simulink model "main"  (R2022a)
settings: Solver=FixedStepDiscrete  StartTime=0.0  StopTime=Inf  FixedStep=(50e-6)-(sim_en*4.995e-5)  RelTol=1e-3  EnableMultiTasking=on
model workspace (MAT data in the model file):
  Param : Simulink.Parameter (value not decoded)
  ac_ok : Simulink.Signal (value not decoded)
  ac_ok_120 : Simulink.Signal (value not decoded)
  bulk_voltage : Simulink.Signal (value not decoded)
  burstduty_integ_max : Simulink.Signal (value not decoded)
  burstduty_integ_min : Simulink.Signal (value not decoded)
  burstduty_ki : Simulink.Signal (value not decoded)
  burstduty_kp : Simulink.Signal (value not decoded)
  calib_ok : Simulink.Signal (value not decoded)
  can_addr1 : Simulink.Signal (value not decoded)
  can_addr2 : Simulink.Signal (value not decoded)
  can_addr3 : Simulink.Signal (value not decoded)
  can_addr4 : Simulink.Signal (value not decoded)
  can_data_rx : Simulink.Signal (value not decoded)
  can_data_tx : Simulink.Signal (value not decoded)
  can_timeout_120 : Simulink.Signal (value not decoded)
  chksum_scircv : Simulink.Signal (value not decoded)
  clllc_en_120 : Simulink.Signal (value not decoded)
  clllc_fault_120 : Simulink.Signal (value not decoded)
  clllc_ok_120 : Simulink.Signal (value not decoded)
  cmpss1h : Simulink.Signal (value not decoded)
  cmpss1l : Simulink.Signal (value not decoded)
  cmpss2h : Simulink.Signal (value not decoded)
  cmpss2l : Simulink.Signal (value not decoded)
  cmpss3h : Simulink.Signal (value not decoded)
  cmpss3l : Simulink.Signal (value not decoded)
  cmpss4h : Simulink.Signal (value not decoded)
  cmpss4l : Simulink.Signal (value not decoded)
  cmpss5h : Simulink.Signal (value not decoded)
  cmpss5l : Simulink.Signal (value not decoded)
  cmpss6h : Simulink.Signal (value not decoded)
  cmpss6l : Simulink.Signal (value not decoded)
  cmpss7h : Simulink.Signal (value not decoded)
  cmpss7l : Simulink.Signal (value not decoded)
  cmpss8h : Simulink.Signal (value not decoded)
  cmpss8l : Simulink.Signal (value not decoded)
  cnt_idle : Simulink.Signal (value not decoded)
  cnt_orps : Simulink.Signal (value not decoded)
  cnt_scircv : Simulink.Signal (value not decoded)
  cnt_scixmt : Simulink.Signal (value not decoded)
  cnt_scixmt_func : Simulink.Signal (value not decoded)
  cnt_temp_mux : Simulink.Signal (value not decoded)
  cnt_vdroop : Simulink.Signal (value not decoded)
  config_ok : Simulink.Signal (value not decoded)
  control_en : Simulink.Signal (value not decoded)
  cp_ready_120 : Simulink.Signal (value not decoded)
  d2d_en : Simulink.Signal (value not decoded)
  dchg_off : Simulink.Signal (value not decoded)
  debug_dacb : Simulink.Signal (value not decoded)
  debug_dacc : Simulink.Signal (value not decoded)
  debug_msg1 : Simulink.Signal (value not decoded)
  debug_msg2 : Simulink.Signal (value not decoded)
  debug_msg3 : Simulink.Signal (value not decoded)
  debug_msg4 : Simulink.Signal (value not decoded)
  debug_msg5 : Simulink.Signal (value not decoded)
  debug_msg6 : Simulink.Signal (value not decoded)
  dir_v2g : Simulink.Signal (value not decoded)
  eoss_llc1 : Simulink.Signal (value not decoded)
  eoss_llc2 : Simulink.Signal (value not decoded)
  eoss_orps : Simulink.Signal (value not decoded)
  fault_ocp : Simulink.Signal (value not decoded)
  fault_otp : Simulink.Signal (value not decoded)
  fault_ovp : Simulink.Signal (value not decoded)
  fut_en : Simulink.Signal (value not decoded)
  fwd_en_120 : Simulink.Signal (value not decoded)
  gain_llc1_sec_idc : Simulink.Signal (value not decoded)
  gain_llc1_temp_sr : Simulink.Signal (value not decoded)
  gain_llc2_sec_idc : Simulink.Signal (value not decoded)
  gain_vbat : Simulink.Signal (value not decoded)
  gain_vbulk : Simulink.Signal (value not decoded)
  gain_vout : Simulink.Signal (value not decoded)
  input_current_phasea : Simulink.Signal (value not decoded)
  input_current_phaseb : Simulink.Signal (value not decoded)
  input_current_phasec : Simulink.Signal (value not decoded)
  input_freq : Simulink.Signal (value not decoded)
  input_power : Simulink.Signal (value not decoded)
  input_voltage_phasea : Simulink.Signal (value not decoded)
  input_voltage_phaseb : Simulink.Signal (value not decoded)
  input_voltage_phasec : Simulink.Signal (value not decoded)
  ishare_arbiter : Simulink.Signal (value not decoded)
  ishare_thresh : Simulink.Signal (value not decoded)
  led_g : Simulink.Signal (value not decoded)
  led_r : Simulink.Signal (value not decoded)
  led_y : Simulink.Signal (value not decoded)
  llc1_burst_integ : Simulink.Signal (value not decoded)
  llc1_burstduty_buffer : Simulink.Signal (value not decoded)
  llc1_pfm_error : Simulink.Signal (value not decoded)
  llc1_pfm_integ : Simulink.Signal (value not decoded)
  llc1_pfm_prop : Simulink.Signal (value not decoded)
  llc1_pri_idc : Simulink.Signal (value not decoded)
  llc1_ps_buffer : Simulink.Signal (value not decoded)
  llc1_pspwm_error : Simulink.Signal (value not decoded)
  llc1_pspwm_integ : Simulink.Signal (value not decoded)
  llc1_pspwm_prop : Simulink.Signal (value not decoded)
  llc1_sec_idc : Simulink.Signal (value not decoded)
  llc1_temp_sr : Simulink.Signal (value not decoded)
  llc1_ts_tbctr_buffer : Simulink.Signal (value not decoded)
  llc2_burst_integ : Simulink.Signal (value not decoded)
  llc2_burstduty_buffer : Simulink.Signal (value not decoded)
  llc2_en : Simulink.Signal (value not decoded)
  llc2_en_buffer : Simulink.Signal (value not decoded)
  llc2_pfm_error : Simulink.Signal (value not decoded)
  llc2_pfm_integ : Simulink.Signal (value not decoded)
  llc2_pfm_prop : Simulink.Signal (value not decoded)
  llc2_pri_idc : Simulink.Signal (value not decoded)
  llc2_ps_buffer : Simulink.Signal (value not decoded)
  llc2_pspwm_error : Simulink.Signal (value not decoded)
  llc2_pspwm_integ : Simulink.Signal (value not decoded)
  llc2_pspwm_prop : Simulink.Signal (value not decoded)
  llc2_sec_idc : Simulink.Signal (value not decoded)
  llc2_temp_sr : Simulink.Signal (value not decoded)
  llc2_ts_tbctr_buffer : Simulink.Signal (value not decoded)
  loop_adcint : Simulink.Signal (value not decoded)
  loop_control : Simulink.Signal (value not decoded)
  loop_idle : Simulink.Signal (value not decoded)
  mid_bulk_voltage : Simulink.Signal (value not decoded)
  mode_120 : Simulink.Signal (value not decoded)
  mode_cc_cv : Simulink.Signal (value not decoded)
  myParam : mpt.Parameter (value not decoded)
  obc_ok_120 : Simulink.Signal (value not decoded)
  offset_llc1_sec_idc : Simulink.Signal (value not decoded)
  offset_llc1_temp_sr : Simulink.Signal (value not decoded)
  offset_llc2_sec_idc : Simulink.Signal (value not decoded)
  offset_vbat : Simulink.Signal (value not decoded)
  offset_vbulk : Simulink.Signal (value not decoded)
  offset_vout : Simulink.Signal (value not decoded)
  openloop_en : Simulink.Signal (value not decoded)
  openloop_fault_en : Simulink.Signal (value not decoded)
  ot_fault_120 : Simulink.Signal (value not decoded)
  pfc_en : Simulink.Signal (value not decoded)
  pfc_en_120 : Simulink.Signal (value not decoded)
  pfc_fw_revision : Simulink.Signal (value not decoded)
  pfc_fw_revision_bootloader : Simulink.Signal (value not decoded)
  pfc_fw_revision_debug : Simulink.Signal (value not decoded)
  pfc_ok : Simulink.Signal (value not decoded)
  pfc_ok_120 : Simulink.Signal (value not decoded)
  pfm_a0 : Simulink.Signal (value not decoded)
  pfm_a1 : Simulink.Signal (value not decoded)
  pfm_integ_max : Simulink.Signal (value not decoded)
  pfm_integ_min : Simulink.Signal (value not decoded)
  pfm_ki : Simulink.Signal (value not decoded)
  pfm_kp : Simulink.Signal (value not decoded)
  pri_fut_en : Simulink.Signal (value not decoded)
  pri_fut_en_buffer : Simulink.Signal (value not decoded)
  pri_halfbridge_en : Simulink.Signal (value not decoded)
  pri_halfbridge_en_buffer : Simulink.Signal (value not decoded)
  pspwm_integ_max : Simulink.Signal (value not decoded)
  pspwm_integ_min : Simulink.Signal (value not decoded)
  pspwm_ki : Simulink.Signal (value not decoded)
  pspwm_kp : Simulink.Signal (value not decoded)
  ref_idclink_max : Simulink.Signal (value not decoded)
  ref_iout : Simulink.Signal (value not decoded)
  ref_iout_calib : Simulink.Signal (value not decoded)
  ref_iout_llc1 : Simulink.Signal (value not decoded)
  ref_iout_llc1_calib : Simulink.Signal (value not decoded)
  ref_iout_llc2 : Simulink.Signal (value not decoded)
  ref_iout_llc2_calib : Simulink.Signal (value not decoded)
  ref_pout : Simulink.Signal (value not decoded)
  ref_ss_llc1 : Simulink.Signal (value not decoded)
  ref_ss_llc2 : Simulink.Signal (value not decoded)
  ref_ss_orps : Simulink.Signal (value not decoded)
  ref_vbat : Simulink.Signal (value not decoded)
  ref_vbat_calib : Simulink.Signal (value not decoded)
  ref_vbulk : Simulink.Signal (value not decoded)
  ref_vbulk_calib : Simulink.Signal (value not decoded)
  ref_vbulk_llc1_calib : Simulink.Signal (value not decoded)
  ref_vbulk_llc2_calib : Simulink.Signal (value not decoded)
  ref_vout : Simulink.Signal (value not decoded)
  ref_vout_calib : Simulink.Signal (value not decoded)
  relay_en : Simulink.Signal (value not decoded)
  reset_flag : Simulink.Signal (value not decoded)
  rev_en_120 : Simulink.Signal (value not decoded)
  runtime_control : Simulink.Signal (value not decoded)
  runtime_idle : Simulink.Signal (value not decoded)
  scircv_buffer : Simulink.Signal (value not decoded)
  scircv_buffer_tmp : Simulink.Signal (value not decoded)
  scircv_buffer_tmp_idx0 : Simulink.Signal (value not decoded)
  scircv_chksum : Simulink.Signal (value not decoded)
  scircv_chksum_ok : Simulink.Signal (value not decoded)
  scircv_parse_ok : Simulink.Signal (value not decoded)
  scixmt_buffer : Simulink.Signal (value not decoded)
  scixmt_chksum : Simulink.Signal (value not decoded)
  scixmt_func : Simulink.Signal (value not decoded)
  scixmt_word0_lsb : Simulink.Signal (value not decoded)
  scixmt_word0_msb : Simulink.Signal (value not decoded)
  scixmt_word1_lsb : Simulink.Signal (value not decoded)
  scixmt_word1_msb : Simulink.Signal (value not decoded)
  scixmt_word2_lsb : Simulink.Signal (value not decoded)
  scixmt_word2_msb : Simulink.Signal (value not decoded)
  scixmt_wr : Simulink.Signal (value not decoded)
  ss_step : Simulink.Signal (value not decoded)
  state_calib : Simulink.Signal (value not decoded)
  state_control : Simulink.Signal (value not decoded)
  state_hkeep : Simulink.Signal (value not decoded)
  status_cmpss : Simulink.Signal (value not decoded)
  status_control : Simulink.Signal (value not decoded)
  status_digin : Simulink.Signal (value not decoded)
  status_digout : Simulink.Signal (value not decoded)
  status_fault : Simulink.Signal (value not decoded)
  status_input : Simulink.Signal (value not decoded)
  status_pfc : Simulink.Signal (value not decoded)
  temp_inlet : Simulink.Signal (value not decoded)
  temp_llc1_fet_hs : Simulink.Signal (value not decoded)
  temp_llc2_fet_hs : Simulink.Signal (value not decoded)
  temp_mux : Simulink.Signal (value not decoded)
  temp_mux_s0 : Simulink.Signal (value not decoded)
  temp_mux_s1 : Simulink.Signal (value not decoded)
  temp_mux_s2 : Simulink.Signal (value not decoded)
  temp_outlet : Simulink.Signal (value not decoded)
  temp_pfc_fet_hsa : Simulink.Signal (value not decoded)
  temp_pfc_fet_hsb : Simulink.Signal (value not decoded)
  temp_pfc_fet_hsc : Simulink.Signal (value not decoded)
  temp_pfc_fet_lsa : Simulink.Signal (value not decoded)
  temp_pfc_fet_lsb : Simulink.Signal (value not decoded)
  temp_pfc_fet_lsc : Simulink.Signal (value not decoded)
  test_mode : Simulink.Signal (value not decoded)
  tfcv_cc : Simulink.Signal (value not decoded)
  tfcv_cc_llc2 : Simulink.Signal (value not decoded)
  tfcv_cv : Simulink.Signal (value not decoded)
  tfcv_sr_en : Simulink.Signal (value not decoded)
  tfv_assert_llc1_pri_idc : Simulink.Signal (value not decoded)
  tfv_assert_llc1_sec_idc : Simulink.Signal (value not decoded)
  tfv_assert_llc1_temp_sr : Simulink.Signal (value not decoded)
  tfv_assert_llc2_pri_idc : Simulink.Signal (value not decoded)
  tfv_assert_llc2_sec_idc : Simulink.Signal (value not decoded)
  tfv_assert_llc2_temp_sr : Simulink.Signal (value not decoded)
  tfv_assert_temp_outlet : Simulink.Signal (value not decoded)
  tfv_assert_vaux_uv : Simulink.Signal (value not decoded)
  tfv_assert_vbat : Simulink.Signal (value not decoded)
  tfv_assert_vbulk : Simulink.Signal (value not decoded)
  tfv_assert_vout : Simulink.Signal (value not decoded)
  tfv_cnt_tz : Simulink.Signal (value not decoded)
  tfv_deassert_llc1_pri_idc : Simulink.Signal (value not decoded)
  tfv_deassert_llc1_sec_idc : Simulink.Signal (value not decoded)
  tfv_deassert_llc1_temp_sr : Simulink.Signal (value not decoded)
  tfv_deassert_llc2_pri_idc : Simulink.Signal (value not decoded)
  tfv_deassert_llc2_sec_idc : Simulink.Signal (value not decoded)
  tfv_deassert_llc2_temp_sr : Simulink.Signal (value not decoded)
  tfv_deassert_temp_outlet : Simulink.Signal (value not decoded)
  tfv_deassert_vaux_uv : Simulink.Signal (value not decoded)
  tfv_deassert_vbat : Simulink.Signal (value not decoded)
  tfv_deassert_vbulk : Simulink.Signal (value not decoded)
  tfv_deassert_vout : Simulink.Signal (value not decoded)
  tfv_llc1_pri_idc : Simulink.Signal (value not decoded)
  tfv_llc1_sec_idc : Simulink.Signal (value not decoded)
  tfv_llc1_temp_sr : Simulink.Signal (value not decoded)
  tfv_llc2_pri_idc : Simulink.Signal (value not decoded)
  tfv_llc2_sec_idc : Simulink.Signal (value not decoded)
  tfv_llc2_temp_sr : Simulink.Signal (value not decoded)
  tfv_temp_outlet : Simulink.Signal (value not decoded)
  tfv_vaux_uv : Simulink.Signal (value not decoded)
  tfv_vbat : Simulink.Signal (value not decoded)
  tfv_vbulk : Simulink.Signal (value not decoded)
  tfv_vout : Simulink.Signal (value not decoded)
  timer_1ms : Simulink.Signal (value not decoded)
  tz : Simulink.Signal (value not decoded)
  valve_en : Simulink.Signal (value not decoded)
  vaux : Simulink.Signal (value not decoded)
  vbat : Simulink.Signal (value not decoded)
  vbulk : Simulink.Signal (value not decoded)
  vout : Simulink.Signal (value not decoded)
undefined symbols (not defined in the file or in its folder): CAN_O_INT, CANA_BASE, Down, GPTRIP1SEL, GPTRIP2SEL, TZ1, TZ2, Up
libraries: hdlsllib x159, simulink x100, c2837xDlib x24, c2807xlib x16, c280xlib x13, c2802xlib x12, canmsglib x8, idelinklib_common x2, c2000lib x1, c281xlib x1
(part 5 of 15)

== system main/Task_Manager/Tmr_1mS/codegen/Task_1mS/GPIO_Handler ==
  function : TriggerPort  TriggerType=function-call  VariantControl=Variant
  Cast{,1..3} (4 alike) : DataTypeConversion  OutDataTypeStr=boolean  SaturateOnIntegerOverflow=off  RndMeth=Floor
  Cast{4..7} (4 alike) : DataTypeConversion  Commented=on  OutDataTypeStr=boolean  SaturateOnIntegerOverflow=off  RndMeth=Floor
  Constant : Constant
  Constant1 : Constant  Commented=on
  Data Store Read1 : DataStoreRead  Commented=on  DataStoreName=pfc_en_120  IndexOptions=Index vector (dialog)  Indices=1  OutputSizes=1
  Data Store Read2 : DataStoreRead  Commented=on  DataStoreName=obc_ok_120  IndexOptions=Index vector (dialog)  Indices=1  OutputSizes=1
  Data Store Read5 : DataStoreRead  Commented=on  DataStoreName=clllc_ok_120  IndexOptions=Index vector (dialog)  Indices=1  OutputSizes=1
  Data Store Write1 : DataStoreWrite  DataStoreName=ac_ok_120  IndexOptions=Index vector (dialog)  Indices=1  OutputSizes=1
  Data Store Write12 : DataStoreWrite  DataStoreName=cp_ready_120  IndexOptions=Index vector (dialog)  Indices=1  OutputSizes=1
  Data Store Write2 : DataStoreWrite  DataStoreName=pfc_ok_120  IndexOptions=Index vector (dialog)  Indices=1  OutputSizes=1
  Data Store Write3 : DataStoreWrite  DataStoreName=clllc_en_120  IndexOptions=Index vector (dialog)  Indices=1  OutputSizes=1
  Digital Input1 : c2837xDlib/Digital Input  Commented=on  GPIO_Number=GPIO56~GPIO63  GPIO_Bit0=off  GPIO_Bit1=off  GPIO_Bit2=off  GPIO_Bit3=off  GPIO_Bit4=on  GPIO_Bit5=off  GPIO_Bit6=off  GPIO_Bit7=off  sampleTime=0.001  dataType=auto  GPIO_Bit0_Qualification=Sync to SYSCLKOUT  GPIO_Bit1_Qualification=Sync to SYSCLKOUT  GPIO_Bit2_Qualification=Sync to SYSCLKOUT  GPIO_Bit3_Qualification=Sync to SYSCLKOUT  GPIO_Bit4_Qualification=Sync to SYSCLKOUT  GPIO_Bit5_Qualification=Sync to SYSCLKOUT  GPIO_Bit6_Qualification=Sync to SYSCLKOUT  GPIO_Bit7_Qualification=Sync to SYSCLKOUT  Qualification_Period=-1
      settings: SourceProductBaseCode=TIC2000
  Digital Input2 : c2837xDlib/Digital Input  Commented=on  GPIO_Number=GPIO56~GPIO63  GPIO_Bit0=off  GPIO_Bit1=off  GPIO_Bit2=off  GPIO_Bit3=on  GPIO_Bit4=off  GPIO_Bit5=off  GPIO_Bit6=off  GPIO_Bit7=off  sampleTime=0.001  dataType=auto  GPIO_Bit0_Qualification=Sync to SYSCLKOUT  GPIO_Bit1_Qualification=Sync to SYSCLKOUT  GPIO_Bit2_Qualification=Sync to SYSCLKOUT  GPIO_Bit3_Qualification=Sync to SYSCLKOUT  GPIO_Bit4_Qualification=Sync to SYSCLKOUT  GPIO_Bit5_Qualification=Sync to SYSCLKOUT  GPIO_Bit6_Qualification=Sync to SYSCLKOUT  GPIO_Bit7_Qualification=Sync to SYSCLKOUT  Qualification_Period=-1
      settings: SourceProductBaseCode=TIC2000
  Digital Input3 : c2837xDlib/Digital Input  Commented=on  GPIO_Number=GPIO56~GPIO63  GPIO_Bit0=off  GPIO_Bit1=on  GPIO_Bit2=off  GPIO_Bit3=off  GPIO_Bit4=off  GPIO_Bit5=off  GPIO_Bit6=off  GPIO_Bit7=off  sampleTime=0.001  dataType=auto  GPIO_Bit0_Qualification=Sync to SYSCLKOUT  GPIO_Bit1_Qualification=Sync to SYSCLKOUT  GPIO_Bit2_Qualification=Sync to SYSCLKOUT  GPIO_Bit3_Qualification=Sync to SYSCLKOUT  GPIO_Bit4_Qualification=Sync to SYSCLKOUT  GPIO_Bit5_Qualification=Sync to SYSCLKOUT  GPIO_Bit6_Qualification=Sync to SYSCLKOUT  GPIO_Bit7_Qualification=Sync to SYSCLKOUT  Qualification_Period=-1
      settings: SourceProductBaseCode=TIC2000
  Digital Input4 : c2837xDlib/Digital Input  Commented=on  GPIO_Number=GPIO56~GPIO63  GPIO_Bit0=off  GPIO_Bit1=off  GPIO_Bit2=on  GPIO_Bit3=off  GPIO_Bit4=off  GPIO_Bit5=off  GPIO_Bit6=off  GPIO_Bit7=off  sampleTime=0.001  dataType=auto  GPIO_Bit0_Qualification=Sync to SYSCLKOUT  GPIO_Bit1_Qualification=Sync to SYSCLKOUT  GPIO_Bit2_Qualification=Sync to SYSCLKOUT  GPIO_Bit3_Qualification=Sync to SYSCLKOUT  GPIO_Bit4_Qualification=Sync to SYSCLKOUT  GPIO_Bit5_Qualification=Sync to SYSCLKOUT  GPIO_Bit6_Qualification=Sync to SYSCLKOUT  GPIO_Bit7_Qualification=Sync to SYSCLKOUT  Qualification_Period=-1
      settings: SourceProductBaseCode=TIC2000
  Digital Output : c2837xDlib/Digital Output  Commented=on  GPIO_Number=GPIO64~GPIO71  GPIO_Bit0=off  GPIO_BIT0_Toggle=off  GPIO_Bit1=off  GPIO_BIT1_Toggle=off  GPIO_Bit2=off  GPIO_BIT2_Toggle=off  GPIO_Bit3=on  GPIO_BIT3_Toggle=off  GPIO_Bit4=off  GPIO_BIT4_Toggle=off  GPIO_Bit5=off  GPIO_BIT5_Toggle=off  GPIO_Bit6=off  GPIO_BIT6_Toggle=off  GPIO_Bit7=off  GPIO_BIT7_Toggle=off
      settings: SourceProductBaseCode=TIC2000
  Digital Output1 : c2837xDlib/Digital Output  Commented=on  GPIO_Number=GPIO64~GPIO71  GPIO_Bit0=off  GPIO_BIT0_Toggle=off  GPIO_Bit1=off  GPIO_BIT1_Toggle=off  GPIO_Bit2=off  GPIO_BIT2_Toggle=off  GPIO_Bit3=off  GPIO_BIT3_Toggle=off  GPIO_Bit4=on  GPIO_BIT4_Toggle=off  GPIO_Bit5=off  GPIO_BIT5_Toggle=off  GPIO_Bit6=off  GPIO_BIT6_Toggle=off  GPIO_Bit7=off  GPIO_BIT7_Toggle=off
      settings: SourceProductBaseCode=TIC2000
  Digital Output2 : c2837xDlib/Digital Output  Commented=on  GPIO_Number=GPIO48~GPIO55  GPIO_Bit0=off  GPIO_BIT0_Toggle=off  GPIO_Bit1=on  GPIO_BIT1_Toggle=off  GPIO_Bit2=off  GPIO_BIT2_Toggle=off  GPIO_Bit3=off  GPIO_BIT3_Toggle=off  GPIO_Bit4=off  GPIO_BIT4_Toggle=off  GPIO_Bit5=off  GPIO_BIT5_Toggle=off  GPIO_Bit6=off  GPIO_BIT6_Toggle=off  GPIO_Bit7=off  GPIO_BIT7_Toggle=off
      settings: SourceProductBaseCode=TIC2000
  Digital Output3 : c2837xDlib/Digital Output  Commented=on  GPIO_Number=GPIO64~GPIO71  GPIO_Bit0=on  GPIO_BIT0_Toggle=off  GPIO_Bit1=off  GPIO_BIT1_Toggle=off  GPIO_Bit2=off  GPIO_BIT2_Toggle=off  GPIO_Bit3=off  GPIO_BIT3_Toggle=off  GPIO_Bit4=off  GPIO_BIT4_Toggle=off  GPIO_Bit5=off  GPIO_BIT5_Toggle=off  GPIO_Bit6=off  GPIO_BIT6_Toggle=off  GPIO_Bit7=off  GPIO_BIT7_Toggle=off
      settings: SourceProductBaseCode=TIC2000
  Update_ACOK : Subsystem
  Update_CLLLCEN : Subsystem
  Update_CPReady : Subsystem
  Update_PFCOK : Subsystem
  wires:
  Cast3/1 -> Update_CLLLCEN/1(Dig_Input)
  Cast/1 -> Update_ACOK/1(Dig_Input)
  Data Store Read5/1 -> Cast5/1
  Cast1/1 -> Update_PFCOK/1(Dig_Input)
  Data Store Read1/1 -> Cast6/1
  Data Store Read2/1 -> Cast4/1
  Update_CLLLCEN/1(Dig_Input_State) -> Data Store Write3/1
  Update_ACOK/1(Dig_Input_State) -> Data Store Write1/1
  Cast2/1 -> Update_CPReady/1(Dig_Input)
  Update_PFCOK/1(Dig_Input_State) -> Data Store Write2/1
  Cast4/1 -> Digital Output2/1
  Cast6/1 -> Digital Output/1
  Cast5/1 -> Digital Output1/1
  Update_CPReady/1(Dig_Input_State) -> Data Store Write12/1
  Cast7/1 -> Digital Output3/1
  Constant1/1 -> Cast7/1
  Constant/1 -> Cast1/1, Cast2/1, Cast3/1, Cast/1  "CP_READY"

== system main/Task_Manager/Tmr_1s/codegen/Task_1S/addressing_temp_mux ==
  note: Note:
      | 0   dec0: llc1_temp_sr
      | 1   dec2: llc2_temp_sr
      | 2   dec6: temp_outlet
  function : TriggerPort  TriggerType=function-call  VariantControl=Variant
  Data Store Read1 : DataStoreRead  DataStoreName=cnt_temp_mux  IndexOptions=Index vector (dialog)  Indices=1  OutputSizes=1
  If : If  IfExpression=u1 == 0  ElseIfExpressions=u1 == 1, u1 == 2
  cnt_temp_mux0 : Subsystem  TreatAsAtomicUnit=on
  cnt_temp_mux1 : Subsystem  TreatAsAtomicUnit=on
  cnt_temp_mux2 : Subsystem  TreatAsAtomicUnit=on
  wires:
  Data Store Read1/1 -> If/1
  If/1 -> cnt_temp_mux0/Action
  If/2 -> cnt_temp_mux1/Action
  If/3 -> cnt_temp_mux2/Action

== system main/Task_Manager/Tmr_1s/codegen/Task_1S/cnt_temp_mux ==
  function : TriggerPort  TriggerType=function-call  VariantControl=Variant
  Data Store Read : DataStoreRead  DataStoreName=cnt_temp_mux  IndexOptions=Index vector (dialog)  Indices=1  OutputSizes=1
  If : If  IfExpression=u1 < 3
  cnt_temp_mux : Subsystem  TreatAsAtomicUnit=on
  cnt_temp_mux_sat : Subsystem  TreatAsAtomicUnit=on
  wires:
  If/2 -> cnt_temp_mux_sat/Action
  Data Store Read/1 -> If/1
  If/1 -> cnt_temp_mux/Action

== system main/Task_Manager/Tmr_20mS/codegen/Task_20mS/Rx_Handler ==
  function : TriggerPort  TriggerType=function-call  VariantControl=Variant
  Data Store Read : DataStoreRead  DataStoreName=b05_MB10Received  IndexOptions=Index vector (dialog)  Indices=1  OutputSizes=1
  Data Store Read1 : DataStoreRead  DataStoreName=b06_MB11Received  IndexOptions=Index vector (dialog)  Indices=1  OutputSizes=1
  Data Store Read2 : DataStoreRead  DataStoreName=b07_MB12Received  IndexOptions=Index vector (dialog)  Indices=1  OutputSizes=1
  If : If  NumInputs=3  IfExpression=u1 == 1  ElseIfExpressions=u2 ==1, u3==1
  ProcessMB10 : Subsystem  TreatAsAtomicUnit=on
  ProcessMB11 : Subsystem  TreatAsAtomicUnit=on
  ProcessMB12 : Subsystem  TreatAsAtomicUnit=on
  wires:
  If/1 -> ProcessMB10/Action
  If/2 -> ProcessMB11/Action
  If/3 -> ProcessMB12/Action
  Data Store Read/1 -> If/1
  Data Store Read1/1 -> If/2
  Data Store Read2/1 -> If/3

== system main/Task_Manager/Tmr_20mS/codegen/Task_20mS/Tx_Handler ==
  "function " : TriggerPort  TriggerType=function-call  VariantControl=Variant
  Constant4 : Constant  Value=10  OutDataTypeStr=uint16
  Data Store Read : DataStoreRead  DataStoreName=u16TxDelayCount  IndexOptions=Index vector (dialog)  Indices=1  OutputSizes=1
  Data Store Write1 : DataStoreWrite  DataStoreName=u16TxDelayCount  IndexOptions=Index vector (dialog)  Indices=1  OutputSizes=1
  If2 : If  NumInputs=2  IfExpression=u1 == u2
  Increment Stored Integer : simulink/Additional Math & Discrete/Additional Math: Increment - Decrement/Increment Stored Integer
  Run Tx Routine : Subsystem  TreatAsAtomicUnit=on
  wires:
  Data Store Read/1 -> Increment Stored Integer/1
  Increment Stored Integer/1 -> If2/1, Data Store Write1/1
  Constant4/1 -> If2/2
  If2/1 -> Run Tx Routine/Action

== system main/Task_Manager/idle/idle_task/comm_npc/comm_npc/COMM_NPC.calcScircvChksum ==
  scircv_buffer : Inport
  f : TriggerPort  TriggerType=function-call  VariantControl=(inherit)
      settings: CopyFcn=Stateflow.SLINSF.SimulinkMan.removeBlockPreDeleteFcn  PreDeleteFcn=Stateflow.SLINSF.SimulinkMan.unsafePredeleteFcn
  For Iterator Subsystem : Subsystem  TreatAsAtomicUnit=on
  wires:
  scircv_buffer/1 -> For Iterator Subsystem/1(scircv_buffer)

== system main/Task_Manager/idle/idle_task/comm_npc/comm_npc/COMM_NPC.calcScixmtChksum ==
  note: Note:
      | byte0 - header
      | byte1 - w/r
      | byte2 - func
      | byte3, byte4 - word0_lsb, word0_msb
      | byte5, byte6 - word1_lsb, word1_msb
      | byte7, byte8 - word2_lsb, word2_msb
      | byte9 - chksum
      | byte10 - 0x00
      | byte11 - terminator
  f : TriggerPort  TriggerType=function-call  VariantControl=(inherit)
      settings: CopyFcn=Stateflow.SLINSF.SimulinkMan.removeBlockPreDeleteFcn  PreDeleteFcn=Stateflow.SLINSF.SimulinkMan.unsafePredeleteFcn
  Function-Call Generator1 : simulink/Ports & Subsystems/Function-Call Generator  sample_time=-1  numberOfIterations=1  DisallowWideOutput=off
  Function-Call Split3 : FunctionCallSplit  NumOutputPorts=2
  calc_chksum : Subsystem  TreatAsAtomicUnit=on
      settings: RTWSystemCode=Inline
  update_scixmt_buffer : Subsystem  TreatAsAtomicUnit=on
      settings: RTWSystemCode=Inline
  wires:
  Function-Call Split3/2 -> calc_chksum/Trigger
  Function-Call Split3/1 -> update_scixmt_buffer/Trigger
  Function-Call Generator1/1 -> Function-Call Split3/1

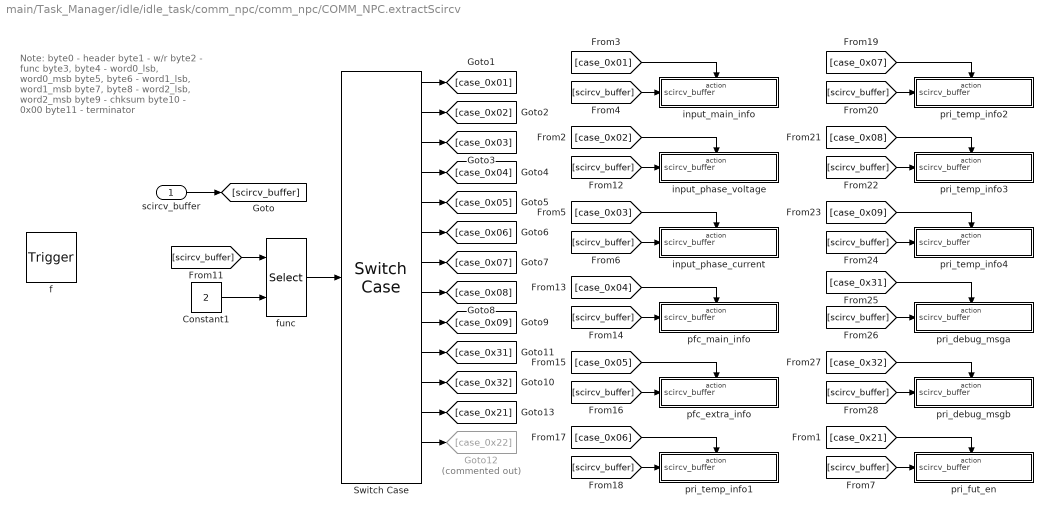
== system main/Task_Manager/idle/idle_task/comm_npc/comm_npc/COMM_NPC.extractScircv ==
  note: Note:
      | byte0 - header
      | byte1 - w/r
      | byte2 - func
      | byte3, byte4 - word0_lsb, word0_msb
      | byte5, byte6 - word1_lsb, word1_msb
      | byte7, byte8 - word2_lsb, word2_msb
      | byte9 - chksum
      | byte10 - 0x00
      | byte11 - terminator
  scircv_buffer : Inport
  f : TriggerPort  TriggerType=function-call  VariantControl=(inherit)
      settings: CopyFcn=Stateflow.SLINSF.SimulinkMan.removeBlockPreDeleteFcn  PreDeleteFcn=Stateflow.SLINSF.SimulinkMan.unsafePredeleteFcn
  Constant1 : Constant  Value=2  OutDataTypeStr=uint8
  Goto12 : Goto  Commented=on  GotoTag=case_0x22
  Switch Case : SwitchCase  CaseConditions={0x01, 0x02, 0x03, 0x04, 0x05, 0x06, 0x07, 0x08, 0x09, 0x31, 0x32, 0x21, 0x22}
  func : Selector  IndexMode=Zero-based  InputPortWidth=12  IndexOptions=Index vector (port)  Indices=[1 3]  OutputSizes=1
  input_main_info : Subsystem  TreatAsAtomicUnit=on
  input_phase_current : Subsystem  TreatAsAtomicUnit=on
  input_phase_voltage : Subsystem  TreatAsAtomicUnit=on
  pfc_extra_info : Subsystem  TreatAsAtomicUnit=on
  pfc_main_info : Subsystem  TreatAsAtomicUnit=on
  pri_debug_msga : Subsystem  TreatAsAtomicUnit=on
  pri_debug_msgb : Subsystem  TreatAsAtomicUnit=on
  pri_fut_en : Subsystem  TreatAsAtomicUnit=on
  pri_temp_info1 : Subsystem  TreatAsAtomicUnit=on
  pri_temp_info2 : Subsystem  TreatAsAtomicUnit=on
  pri_temp_info3 : Subsystem  TreatAsAtomicUnit=on
  pri_temp_info4 : Subsystem  TreatAsAtomicUnit=on
  wires:
  scircv_buffer/1 -> [scircv_buffer]
  Switch Case/7 -> [case_0x07]
  [scircv_buffer] -> pri_temp_info4/1(scircv_buffer)
  [case_0x32] -> pri_debug_msgb/Action
  [scircv_buffer] -> pri_debug_msgb/1(scircv_buffer)
  [case_0x07] -> pri_temp_info2/Action
  Switch Case/2 -> [case_0x02]
  [scircv_buffer] -> pri_temp_info1/1(scircv_buffer)
  Switch Case/11 -> [case_0x32]
  [scircv_buffer] -> pri_debug_msga/1(scircv_buffer)
  [case_0x31] -> pri_debug_msga/Action
  Switch Case/5 -> [case_0x05]
  [scircv_buffer] -> pri_temp_info2/1(scircv_buffer)
  [case_0x08] -> pri_temp_info3/Action
  [scircv_buffer] -> pri_temp_info3/1(scircv_buffer)
  [case_0x06] -> pri_temp_info1/Action
  Switch Case/6 -> [case_0x06]
  [scircv_buffer] -> pfc_main_info/1(scircv_buffer)
  [case_0x02] -> input_phase_voltage/Action
  [case_0x03] -> input_phase_current/Action
  [scircv_buffer] -> input_phase_current/1(scircv_buffer)
  Switch Case/1 -> [case_0x01]
  func/1 -> Switch Case/1
  Switch Case/9 -> [case_0x09]
  [scircv_buffer] -> input_main_info/1(scircv_buffer)
  Constant1/1 -> func/2
  [case_0x09] -> pri_temp_info4/Action
  [case_0x05] -> pfc_extra_info/Action
  Switch Case/3 -> [case_0x03]
  Switch Case/4 -> [case_0x04]
  [case_0x04] -> pfc_main_info/Action
  [scircv_buffer] -> pfc_extra_info/1(scircv_buffer)
  Switch Case/10 -> [case_0x31]
  [scircv_buffer] -> input_phase_voltage/1(scircv_buffer)
  Switch Case/8 -> [case_0x08]
  [scircv_buffer] -> func/1
  [case_0x01] -> input_main_info/Action
  Switch Case/12 -> [case_0x21]
  Switch Case/13 -> Goto12/1
  [scircv_buffer] -> pri_fut_en/1(scircv_buffer)
  [case_0x21] -> pri_fut_en/Action

== system main/Task_Manager/idle/idle_task/comm_npc/comm_npc/COMM_NPC.incrFunc ==
  cnt_scixmt_func : Inport
  f : TriggerPort  TriggerType=function-call  VariantControl=(inherit)
      settings: CopyFcn=Stateflow.SLINSF.SimulinkMan.removeBlockPreDeleteFcn  PreDeleteFcn=Stateflow.SLINSF.SimulinkMan.unsafePredeleteFcn
  Constant10 : Constant  Value=[0, 1, 2, 3, 4, 5, 6, 7, 8, 9, 10, 11]  OutDataTypeStr=uint8
  Constant11 : Constant  Value=[0x1, 0x2, 0x3, 0x4, 0x5, 0x6, 0x7, 0x8, 0x9, 0x31, 0x32, 0x21]  OutDataTypeStr=uint8
  If : If  IfExpression=u1 < 11
  Lookup Table Dynamic : simulink/Lookup Tables/Lookup Table Dynamic  LookUpMeth=Interpolation-Use End Values  OutDataType=fixdt('uint8')  OutScaling=[]  OutputDataTypeScalingMode=Specify via dialog  OutDataTypeStr=uint8  DoSatur=off
  Merge : Merge
  increment : Subsystem  TreatAsAtomicUnit=on
  saturation : Subsystem  TreatAsAtomicUnit=on
  scixmt_func : Outport
  wires:
  If/1 -> increment/Action
  If/2 -> saturation/Action
  cnt_scixmt_func/1 -> If/1
  increment/1(Out1) -> Merge/1
  saturation/1(Out1) -> Merge/2
  Constant10/1 -> Lookup Table Dynamic/2
  Constant11/1 -> Lookup Table Dynamic/3
  Merge/1 -> Lookup Table Dynamic/1
  Lookup Table Dynamic/1 -> scixmt_func/1

== system main/Task_Manager/idle/idle_task/comm_npc/comm_npc/COMM_NPC.packScixmt ==
  note: Note:
      | byte0 - header
      | byte1 - w/r
      | byte2 - func
      | byte3, byte4 - word0_lsb, word0_msb
      | byte5, byte6 - word1_lsb, word1_msb
      | byte7, byte8 - word2_lsb, word2_msb
      | byte9 - chksum
      | byte10 - 0x00
      | byte11 - terminator
  scixmt_chksum : Inport
  f : TriggerPort  TriggerType=function-call  VariantControl=(inherit)
      settings: CopyFcn=Stateflow.SLINSF.SimulinkMan.removeBlockPreDeleteFcn  PreDeleteFcn=Stateflow.SLINSF.SimulinkMan.unsafePredeleteFcn
  Assignment1 : Assignment  IndexMode=Zero-based  DiagnosticForDimensions=Warning  IndexOptions=Index vector (port)  Indices=1  OutputSizes=1
  Assignment2 : Assignment  IndexMode=Zero-based  DiagnosticForDimensions=Warning  IndexOptions=Index vector (port)  Indices=1  OutputSizes=1
  Assignment9 : Assignment  IndexMode=Zero-based  DiagnosticForDimensions=Warning  IndexOptions=Index vector (port)  Indices=1  OutputSizes=1
  Constant : Constant  Value=10  OutDataTypeStr=uint8
  Constant1 : Constant  Value=11  OutDataTypeStr=uint8
  Constant2 : Constant  Value=100  OutDataTypeStr=uint8
  Constant3 : Constant  Value=0  OutDataTypeStr=uint8
  Constant8 : Constant  Value=9  OutDataTypeStr=uint8
  Data Store Read : DataStoreRead  DataStoreName=scixmt_buffer  IndexOptions=Index vector (dialog)  Indices=1  OutputSizes=1
  Data Store Read1 : DataStoreRead  DataStoreName=scixmt_buffer  IndexOptions=Index vector (dialog)  Indices=1  OutputSizes=1
  Data Store Read8 : DataStoreRead  DataStoreName=scixmt_buffer  IndexOptions=Index vector (dialog)  Indices=1  OutputSizes=1
  Data Store Write : DataStoreWrite  DataStoreName=scixmt_buffer  IndexOptions=Index vector (dialog)  Indices=1  OutputSizes=1
  Data Store Write1 : DataStoreWrite  DataStoreName=scixmt_buffer  IndexOptions=Index vector (dialog)  Indices=1  OutputSizes=1
  Data Store Write8 : DataStoreWrite  DataStoreName=scixmt_buffer  IndexOptions=Index vector (dialog)  Indices=1  OutputSizes=1
  wires:
  Constant/1 -> Assignment1/3
  Constant1/1 -> Assignment2/3
  Data Store Read1/1 -> Assignment2/1
  Constant8/1 -> Assignment9/3
  Assignment2/1 -> Data Store Write1/1
  Data Store Read/1 -> Assignment1/1
  Constant2/1 -> Assignment2/2
  Assignment1/1 -> Data Store Write/1
  Assignment9/1 -> Data Store Write8/1
  scixmt_chksum/1 -> Assignment9/2
  Constant3/1 -> Assignment1/2
  Data Store Read8/1 -> Assignment9/1

== system main/Task_Manager/idle/idle_task/comm_npc/comm_npc/COMM_NPC.parseScircv ==
  scircv_buffer_tmp : Inport
  f : TriggerPort  TriggerType=function-call  VariantControl=(inherit)
      settings: CopyFcn=Stateflow.SLINSF.SimulinkMan.removeBlockPreDeleteFcn  PreDeleteFcn=Stateflow.SLINSF.SimulinkMan.unsafePredeleteFcn
  For Iterator Subsystem : Subsystem  TreatAsAtomicUnit=on
  scircv_parse_ok : Outport  InitialOutput=[0]
  wires:
  For Iterator Subsystem/1(scircv_parse_ok) -> scircv_parse_ok/1
  scircv_buffer_tmp/1 -> For Iterator Subsystem/1(scircv_buffer_tmp)

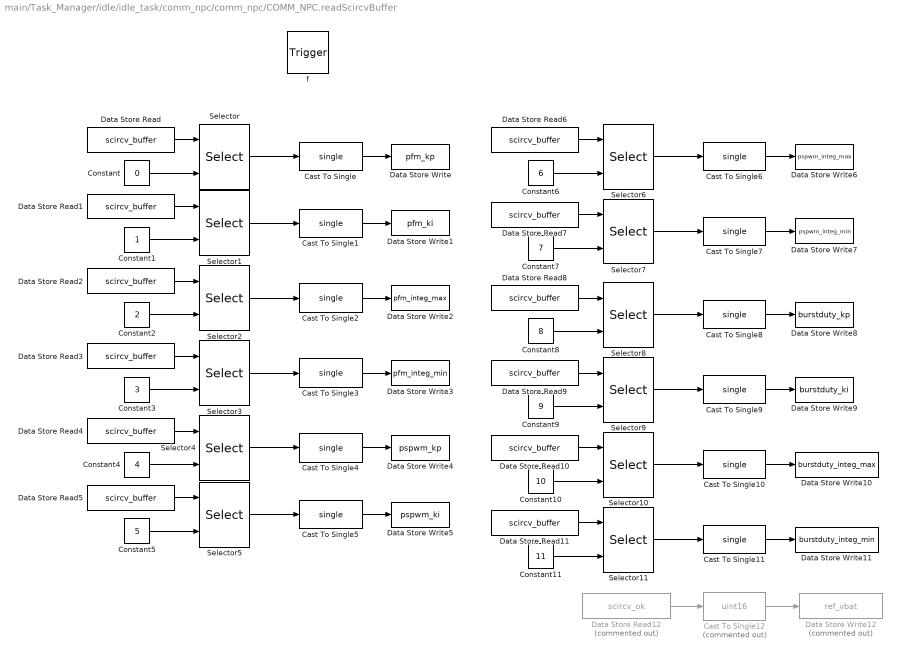
== system main/Task_Manager/idle/idle_task/comm_npc/comm_npc/COMM_NPC.readScircvBuffer ==
  f : TriggerPort  TriggerType=function-call  VariantControl=(inherit)
      settings: CopyFcn=Stateflow.SLINSF.SimulinkMan.removeBlockPreDeleteFcn  PreDeleteFcn=Stateflow.SLINSF.SimulinkMan.unsafePredeleteFcn
  Cast To Single{,1..11} (12 alike) : DataTypeConversion  OutDataTypeStr=single  SaturateOnIntegerOverflow=off  RndMeth=Floor
  Cast To Single12 : DataTypeConversion  Commented=on  OutDataTypeStr=uint16  SaturateOnIntegerOverflow=off  RndMeth=Floor
  Constant : Constant  Value=0  OutDataTypeStr=uint8
  Constant1 : Constant  OutDataTypeStr=uint8
  Constant10 : Constant  Value=10  OutDataTypeStr=uint8
  Constant11 : Constant  Value=11  OutDataTypeStr=uint8
  Constant2 : Constant  Value=2  OutDataTypeStr=uint8
  Constant3 : Constant  Value=3  OutDataTypeStr=uint8
  Constant4 : Constant  Value=4  OutDataTypeStr=uint8
  Constant5 : Constant  Value=5  OutDataTypeStr=uint8
  Constant6 : Constant  Value=6  OutDataTypeStr=uint8
  Constant7 : Constant  Value=7  OutDataTypeStr=uint8
  Constant8 : Constant  Value=8  OutDataTypeStr=uint8
  Constant9 : Constant  Value=9  OutDataTypeStr=uint8
  Data Store Read{,1..11} (12 alike) : DataStoreRead  DataStoreName=scircv_buffer  IndexOptions=Index vector (dialog)  Indices=1  OutputSizes=1
  Data Store Read12 : DataStoreRead  Commented=on  DataStoreName=scircv_ok  IndexOptions=Index vector (dialog)  Indices=1  OutputSizes=1
  Data Store Write : DataStoreWrite  DataStoreName=pfm_kp  IndexOptions=Index vector (dialog)  Indices=1  OutputSizes=1
  Data Store Write1 : DataStoreWrite  DataStoreName=pfm_ki  IndexOptions=Index vector (dialog)  Indices=1  OutputSizes=1
  Data Store Write10 : DataStoreWrite  DataStoreName=burstduty_integ_max  IndexOptions=Index vector (dialog)  Indices=1  OutputSizes=1
  Data Store Write11 : DataStoreWrite  DataStoreName=burstduty_integ_min  IndexOptions=Index vector (dialog)  Indices=1  OutputSizes=1
  Data Store Write12 : DataStoreWrite  Commented=on  DataStoreName=ref_vbat  IndexOptions=Index vector (dialog)  Indices=1  OutputSizes=1
  Data Store Write2 : DataStoreWrite  DataStoreName=pfm_integ_max  IndexOptions=Index vector (dialog)  Indices=1  OutputSizes=1
  Data Store Write3 : DataStoreWrite  DataStoreName=pfm_integ_min  IndexOptions=Index vector (dialog)  Indices=1  OutputSizes=1
  Data Store Write4 : DataStoreWrite  DataStoreName=pspwm_kp  IndexOptions=Index vector (dialog)  Indices=1  OutputSizes=1
  Data Store Write5 : DataStoreWrite  DataStoreName=pspwm_ki  IndexOptions=Index vector (dialog)  Indices=1  OutputSizes=1
  Data Store Write6 : DataStoreWrite  DataStoreName=pspwm_integ_max  IndexOptions=Index vector (dialog)  Indices=1  OutputSizes=1
  Data Store Write7 : DataStoreWrite  DataStoreName=pspwm_integ_min  IndexOptions=Index vector (dialog)  Indices=1  OutputSizes=1
  Data Store Write8 : DataStoreWrite  DataStoreName=burstduty_kp  IndexOptions=Index vector (dialog)  Indices=1  OutputSizes=1
  Data Store Write9 : DataStoreWrite  DataStoreName=burstduty_ki  IndexOptions=Index vector (dialog)  Indices=1  OutputSizes=1
  Selector{,1..11} (12 alike) : Selector  IndexMode=Zero-based  InputPortWidth=12  IndexOptions=Index vector (port)  Indices=[1 3]  OutputSizes=1
  wires:
  Cast To Single/1 -> Data Store Write/1
  Selector/1 -> Cast To Single/1
  Data Store Read/1 -> Selector/1
  Constant/1 -> Selector/2
  Constant1/1 -> Selector1/2
  Data Store Read1/1 -> Selector1/1
  Selector1/1 -> Cast To Single1/1
  Cast To Single1/1 -> Data Store Write1/1
  Cast To Single2/1 -> Data Store Write2/1
  Selector2/1 -> Cast To Single2/1
  Data Store Read2/1 -> Selector2/1
  Constant2/1 -> Selector2/2
  Constant3/1 -> Selector3/2
  Data Store Read3/1 -> Selector3/1
  Selector3/1 -> Cast To Single3/1
  Cast To Single3/1 -> Data Store Write3/1
  Cast To Single7/1 -> Data Store Write7/1
  Selector7/1 -> Cast To Single7/1
  Data Store Read7/1 -> Selector7/1
  Constant7/1 -> Selector7/2
  Constant6/1 -> Selector6/2
  Data Store Read6/1 -> Selector6/1
  Selector6/1 -> Cast To Single6/1
  Cast To Single6/1 -> Data Store Write6/1
  Cast To Single5/1 -> Data Store Write5/1
  Selector5/1 -> Cast To Single5/1
  Data Store Read5/1 -> Selector5/1
  Constant5/1 -> Selector5/2
  Constant4/1 -> Selector4/2
  Data Store Read4/1 -> Selector4/1
  Selector4/1 -> Cast To Single4/1
  Cast To Single4/1 -> Data Store Write4/1
  Cast To Single8/1 -> Data Store Write8/1
  Selector8/1 -> Cast To Single8/1
  Data Store Read8/1 -> Selector8/1
  Constant8/1 -> Selector8/2
  Constant9/1 -> Selector9/2
  Data Store Read9/1 -> Selector9/1
  Selector9/1 -> Cast To Single9/1
  Cast To Single9/1 -> Data Store Write9/1
  Cast To Single11/1 -> Data Store Write11/1
  Selector11/1 -> Cast To Single11/1
  Data Store Read11/1 -> Selector11/1
  Constant11/1 -> Selector11/2
  Constant10/1 -> Selector10/2
  Data Store Read10/1 -> Selector10/1
  Selector10/1 -> Cast To Single10/1
  Cast To Single10/1 -> Data Store Write10/1
  Data Store Read12/1 -> Cast To Single12/1
  Cast To Single12/1 -> Data Store Write12/1

== system main/Task_Manager/idle/idle_task/comm_npc/comm_npc/COMM_NPC.readScircvBuffer1 ==
  f : TriggerPort  TriggerType=function-call  VariantControl=(inherit)
      settings: CopyFcn=Stateflow.SLINSF.SimulinkMan.removeBlockPreDeleteFcn  PreDeleteFcn=Stateflow.SLINSF.SimulinkMan.unsafePredeleteFcn
  Cast To Single{,1..7} (8 alike) : DataTypeConversion  OutDataTypeStr=single  SaturateOnIntegerOverflow=off  RndMeth=Floor
  Cast To Single8 : DataTypeConversion  Commented=on  OutDataTypeStr=single  SaturateOnIntegerOverflow=off  RndMeth=Floor
  Constant2 : Constant  Value=9  OutDataTypeStr=uint8
  Data Store Read : DataStoreRead  DataStoreName=scircv_buffer  IndexOptions=Index vector (dialog)  Indices=1  OutputSizes=1
  Data Store Read1 : DataStoreRead  DataStoreName=scircv_parse_ok  IndexOptions=Index vector (dialog)  Indices=1  OutputSizes=1
  Data Store Read2 : DataStoreRead  DataStoreName=input_freq  IndexOptions=Index vector (dialog)  Indices=1  OutputSizes=1
  Data Store Read3 : DataStoreRead  DataStoreName=input_voltage_phaseb  IndexOptions=Index vector (dialog)  Indices=1  OutputSizes=1
  Data Store Read4 : DataStoreRead  DataStoreName=scircv_chksum_ok  IndexOptions=Index vector (dialog)  Indices=1  OutputSizes=1
  Data Store Read5 : DataStoreRead  DataStoreName=scircv_chksum  IndexOptions=Index vector (dialog)  Indices=1  OutputSizes=1
  Data Store Read6 : DataStoreRead  DataStoreName=scixmt_func  IndexOptions=Index vector (dialog)  Indices=1  OutputSizes=1
  Data Store Read7 : DataStoreRead  DataStoreName=ref_pout  IndexOptions=Index vector (dialog)  Indices=1  OutputSizes=1
  Data Store Read8 : DataStoreRead  Commented=on  DataStoreName=cnt_scixmt  IndexOptions=Index vector (dialog)  Indices=1  OutputSizes=1
  Data Store Write1 : DataStoreWrite  DataStoreName=pfm_integ_max  IndexOptions=Index vector (dialog)  Indices=1  OutputSizes=1
  Data Store Write2 : DataStoreWrite  DataStoreName=pfm_kp  IndexOptions=Index vector (dialog)  Indices=1  OutputSizes=1
  Data Store Write3 : DataStoreWrite  DataStoreName=pfm_ki  IndexOptions=Index vector (dialog)  Indices=1  OutputSizes=1
  Data Store Write4 : DataStoreWrite  DataStoreName=pfm_integ_min  IndexOptions=Index vector (dialog)  Indices=1  OutputSizes=1
  Data Store Write5 : DataStoreWrite  DataStoreName=pspwm_kp  IndexOptions=Index vector (dialog)  Indices=1  OutputSizes=1
  Data Store Write6 : DataStoreWrite  DataStoreName=pspwm_ki  IndexOptions=Index vector (dialog)  Indices=1  OutputSizes=1
  Data Store Write7 : DataStoreWrite  DataStoreName=pspwm_integ_max  IndexOptions=Index vector (dialog)  Indices=1  OutputSizes=1
  Data Store Write8 : DataStoreWrite  DataStoreName=pspwm_integ_min  IndexOptions=Index vector (dialog)  Indices=1  OutputSizes=1
  Data Store Write9 : DataStoreWrite  Commented=on  DataStoreName=burstduty_kp  IndexOptions=Index vector (dialog)  Indices=1  OutputSizes=1
  Selector : Selector  IndexMode=Zero-based  InputPortWidth=12  IndexOptions=Index vector (port)  Indices=[1 3]  OutputSizes=1
  wires:
  Data Store Read2/1 -> Cast To Single/1
  Data Store Read3/1 -> Cast To Single1/1
  Cast To Single/1 -> Data Store Write2/1
  Cast To Single1/1 -> Data Store Write3/1
  Data Store Read1/1 -> Cast To Single2/1
  Cast To Single2/1 -> Data Store Write1/1
  Cast To Single3/1 -> Data Store Write4/1
  Data Store Read4/1 -> Cast To Single3/1
  Cast To Single4/1 -> Data Store Write5/1
  Cast To Single5/1 -> Data Store Write6/1
  Constant2/1 -> Selector/2
  Data Store Read/1 -> Selector/1
  Selector/1 -> Cast To Single5/1
  Data Store Read5/1 -> Cast To Single4/1
  Cast To Single6/1 -> Data Store Write7/1
  Data Store Read6/1 -> Cast To Single6/1
  Data Store Read7/1 -> Cast To Single7/1
  Cast To Single7/1 -> Data Store Write8/1
  Cast To Single8/1 -> Data Store Write9/1
  Data Store Read8/1 -> Cast To Single8/1

== system main/Task_Manager/idle/idle_task/comm_npc/comm_npc/COMM_NPC.sendScixmt ==
  scixmt_buffer : Inport  OutDataTypeStr=uint8
  cnt_scixmt : Inport  Port=2  OutDataTypeStr=uint8
  f : TriggerPort  TriggerType=function-call  VariantControl=(inherit)
      settings: CopyFcn=Stateflow.SLINSF.SimulinkMan.removeBlockPreDeleteFcn  PreDeleteFcn=Stateflow.SLINSF.SimulinkMan.unsafePredeleteFcn
  SCI Transmit1 : c280xlib/SCI Transmit  sciModule=A  dataHead=''  dataTail=''  blockingMode=on  outputStatus=off
  Selector : Selector  IndexMode=Zero-based  InputPortWidth=12  IndexOptions=Index vector (port)  Indices=[1 2]  OutputSizes=1
  wires:
  Selector/1 -> SCI Transmit1/1
  scixmt_buffer/1 -> Selector/1
  cnt_scixmt/1 -> Selector/2

== system main/Task_Manager/idle/idle_task/comm_npc/comm_npc/COMM_NPC.verifyScircvChksum ==
  scircv_chksum : Inport
  f : TriggerPort  TriggerType=function-call  VariantControl=(inherit)
      settings: CopyFcn=Stateflow.SLINSF.SimulinkMan.removeBlockPreDeleteFcn  PreDeleteFcn=Stateflow.SLINSF.SimulinkMan.unsafePredeleteFcn
  Constant2 : Constant  Value=9  OutDataTypeStr=uint8
  Data Store Read : DataStoreRead  DataStoreName=scircv_buffer  IndexOptions=Index vector (dialog)  Indices=1  OutputSizes=1
  If : If  NumInputs=2  IfExpression=u1 == u2
  If Action Subsystem : Subsystem  TreatAsAtomicUnit=on
  If Action Subsystem1 : Subsystem  TreatAsAtomicUnit=on
  Merge : Merge
  Selector : Selector  IndexMode=Zero-based  InputPortWidth=12  IndexOptions=Index vector (port)  Indices=[1 3]  OutputSizes=1
  scircv_chksum_ok : Outport  OutDataTypeStr=boolean  InitialOutput=[0]
  wires:
  Merge/1 -> scircv_chksum_ok/1
  If Action Subsystem1/1(Outport) -> Merge/2
  If/2 -> If Action Subsystem1/Action
  Selector/1 -> If/2
  Constant2/1 -> Selector/2
  Data Store Read/1 -> Selector/1
  If Action Subsystem/1(Outport) -> Merge/1
  If/1 -> If Action Subsystem/Action
  scircv_chksum/1 -> If/1

== system main/Task_Manager/idle/idle_task/debug_uart1/control_en ==
  idx : Inport
  Action Port : ActionPort
  Add1 : Sum  AccumDataTypeStr=uint32  OutDataTypeStr=uint32
  Bit Shift1 : hdlsllib/Logic and Bit Operations/Bit Shift  mode=Shift Left Logical  N=16
  Data Store Read2 : DataStoreRead  DataStoreName=control_en  IndexOptions=Index vector (dialog)  Indices=1  OutputSizes=1
  Data Type Conversion1 : DataTypeConversion  OutDataTypeStr=uint32  SaturateOnIntegerOverflow=off  RndMeth=Floor
  Data Type Conversion2 : DataTypeConversion  OutDataTypeStr=uint32  SaturateOnIntegerOverflow=off  RndMeth=Floor
  Rate Transition2 : RateTransition  Integrity=off  Deterministic=off
  Out1 : Outport  VectorParamsAs1DForOutWhenUnconnected=off
  wires:
  Add1/1 -> Out1/1
  idx/1 -> Data Type Conversion1/1
  Bit Shift1/1 -> Add1/1
  Data Type Conversion2/1 -> Add1/2
  Data Type Conversion1/1 -> Bit Shift1/1
  Data Store Read2/1 -> Rate Transition2/1
  Rate Transition2/1 -> Data Type Conversion2/1

== system main/Task_Manager/idle/idle_task/debug_uart1/default ==
  Action Port : ActionPort
  Add1 : Sum  AccumDataTypeStr=uint32  OutDataTypeStr=uint32
  Bit Shift1 : hdlsllib/Logic and Bit Operations/Bit Shift  mode=Shift Left Logical  N=16
  Constant : Constant  Value=19  OutDataTypeStr=uint16  SampleTime=Inf
  Constant1 : Constant  Value=60  OutDataTypeStr=uint16  SampleTime=Inf
  Data Type Conversion1 : DataTypeConversion  OutDataTypeStr=uint32  SaturateOnIntegerOverflow=off  RndMeth=Floor
  Data Type Conversion2 : DataTypeConversion  OutDataTypeStr=uint32  SaturateOnIntegerOverflow=off  RndMeth=Floor
  Out1 : Outport  VectorParamsAs1DForOutWhenUnconnected=off
  wires:
  Add1/1 -> Out1/1
  Constant1/1 -> Data Type Conversion1/1
  Bit Shift1/1 -> Add1/1
  Data Type Conversion2/1 -> Add1/2
  Data Type Conversion1/1 -> Bit Shift1/1
  Constant/1 -> Data Type Conversion2/1

== system main/Task_Manager/idle/idle_task/debug_uart1/llc1_burstduty_tbctr ==
  Inport : Inport
  Action Port : ActionPort
  Add2 : Sum  AccumDataTypeStr=uint32  OutDataTypeStr=uint32
  Bit Shift3 : hdlsllib/Logic and Bit Operations/Bit Shift  mode=Shift Left Logical  N=16
  Data Store Read2 : DataStoreRead  DataStoreName=llc1_burstduty  IndexOptions=Index vector (dialog)  Indices=1  OutputSizes=1
  Data Type Conversion1 : DataTypeConversion  OutDataTypeStr=uint32  SaturateOnIntegerOverflow=off  RndMeth=Floor
  Data Type Conversion4 : DataTypeConversion  OutDataTypeStr=uint32  SaturateOnIntegerOverflow=off  RndMeth=Floor
  Gain : Gain  Gain=100
  Rate Transition2 : RateTransition  Integrity=off  Deterministic=off
  Outport : Outport
  wires:
  Gain/1 -> Data Type Conversion4/1
  Inport/1 -> Data Type Conversion1/1
  Bit Shift3/1 -> Add2/1
  Data Type Conversion4/1 -> Add2/2
  Add2/1 -> Outport/1
  Data Type Conversion1/1 -> Bit Shift3/1
  Data Store Read2/1 -> Rate Transition2/1
  Rate Transition2/1 -> Gain/1

== system main/Task_Manager/idle/idle_task/debug_uart1/llc1_ipri ==
  idx : Inport
  Action Port : ActionPort
  Add1 : Sum  AccumDataTypeStr=uint32  OutDataTypeStr=uint32
  Bit Shift1 : hdlsllib/Logic and Bit Operations/Bit Shift  mode=Shift Left Logical  N=16
  Data Store Read2 : DataStoreRead  DataStoreName=llc1_pri_idc  IndexOptions=Index vector (dialog)  Indices=1  OutputSizes=1
  Data Type Conversion1 : DataTypeConversion  OutDataTypeStr=uint32  SaturateOnIntegerOverflow=off  RndMeth=Floor
  Data Type Conversion2 : DataTypeConversion  OutDataTypeStr=uint32  SaturateOnIntegerOverflow=off  RndMeth=Floor
  Rate Transition2 : RateTransition  Integrity=off  Deterministic=off
  Out1 : Outport  VectorParamsAs1DForOutWhenUnconnected=off
  wires:
  Add1/1 -> Out1/1
  idx/1 -> Data Type Conversion1/1
  Bit Shift1/1 -> Add1/1
  Data Type Conversion2/1 -> Add1/2
  Data Type Conversion1/1 -> Bit Shift1/1
  Rate Transition2/1 -> Data Type Conversion2/1
  Data Store Read2/1 -> Rate Transition2/1

== system main/Task_Manager/idle/idle_task/debug_uart1/llc1_isec ==
  idx : Inport
  Action Port : ActionPort
  Add1 : Sum  AccumDataTypeStr=uint32  OutDataTypeStr=uint32
  Bit Shift1 : hdlsllib/Logic and Bit Operations/Bit Shift  mode=Shift Left Logical  N=16
  Data Store Read2 : DataStoreRead  DataStoreName=llc1_sec_idc  IndexOptions=Index vector (dialog)  Indices=1  OutputSizes=1
  Data Type Conversion1 : DataTypeConversion  OutDataTypeStr=uint32  SaturateOnIntegerOverflow=off  RndMeth=Floor
  Data Type Conversion2 : DataTypeConversion  OutDataTypeStr=uint32  SaturateOnIntegerOverflow=off  RndMeth=Floor
  Rate Transition2 : RateTransition  Integrity=off  Deterministic=off
  Out1 : Outport  VectorParamsAs1DForOutWhenUnconnected=off
  wires:
  Data Store Read2/1 -> Rate Transition2/1
  Rate Transition2/1 -> Data Type Conversion2/1
  Data Type Conversion1/1 -> Bit Shift1/1
  Data Type Conversion2/1 -> Add1/2
  Bit Shift1/1 -> Add1/1
  idx/1 -> Data Type Conversion1/1
  Add1/1 -> Out1/1

== system main/Task_Manager/idle/idle_task/debug_uart1/llc1_period_tbctr ==
  Inport : Inport
  Action Port : ActionPort
  Add2 : Sum  AccumDataTypeStr=uint32  OutDataTypeStr=uint32
  Bit Shift3 : hdlsllib/Logic and Bit Operations/Bit Shift  mode=Shift Left Logical  N=16
  Data Store Read2 : DataStoreRead  DataStoreName=llc1_ts_tbctr  IndexOptions=Index vector (dialog)  Indices=1  OutputSizes=1
  Data Type Conversion1 : DataTypeConversion  OutDataTypeStr=uint32  SaturateOnIntegerOverflow=off  RndMeth=Floor
  Data Type Conversion4 : DataTypeConversion  OutDataTypeStr=uint32  SaturateOnIntegerOverflow=off  RndMeth=Floor
  Rate Transition2 : RateTransition  Integrity=off  Deterministic=off
  Outport : Outport
  wires:
  Rate Transition2/1 -> Data Type Conversion4/1
  Data Store Read2/1 -> Rate Transition2/1
  Data Type Conversion1/1 -> Bit Shift3/1
  Add2/1 -> Outport/1
  Data Type Conversion4/1 -> Add2/2
  Bit Shift3/1 -> Add2/1
  Inport/1 -> Data Type Conversion1/1
